simulink library "INT_Rail_SetPoint"  (R2016b)
settings: Solver=VariableStepAuto  StartTime=0.0  StopTime=10.0  RelTol=1e-3
settings Model: Creator=dulinggang  LastModifiedBy=dulinggang

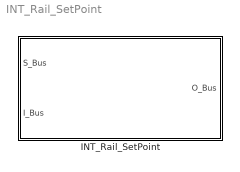
== system INT_Rail_SetPoint ==
  INT_Rail_SetPoint : Subsystem

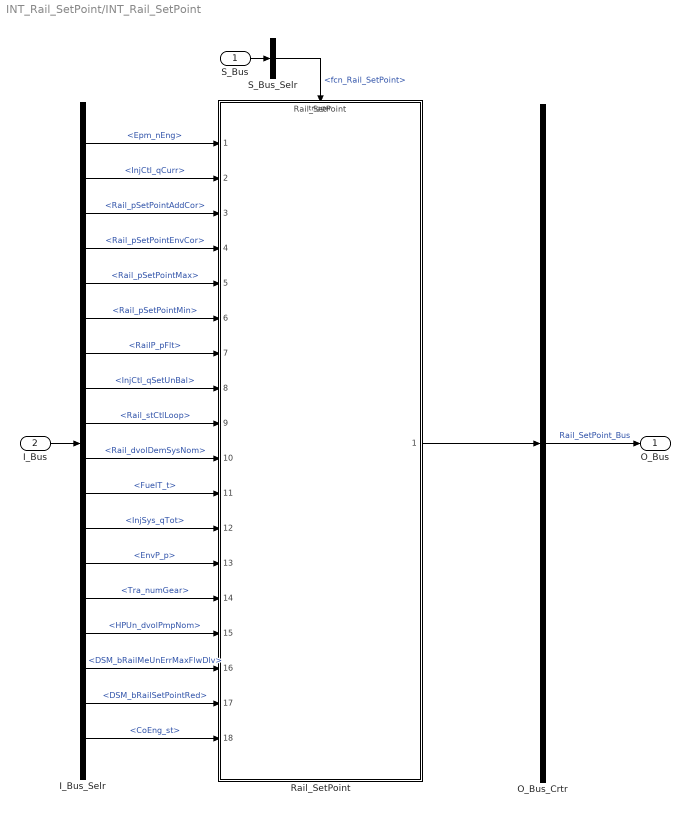
== system INT_Rail_SetPoint/INT_Rail_SetPoint ==
  S_Bus : Inport
  I_Bus : Inport  Port=2
  I_Bus_Selr : BusSelector  OutputSignals=Epm_nEng,InjCtl_qCurr,Rail_pSetPointAddCor,Rail_pSetPointEnvCor,Rail_pSetPointMax,Rail_pSetPointMin,RailP_pFlt,InjCtl_qSetUnBal,Rail_stCtlLoop,Rail_dvolDemSysNom,FuelT_t,InjSys_qTot,EnvP_p,Tra_numGear,HPUn_dvolPmpNom,DSM_bRailMeUnErrMaxFlwDlv,DSM_bRailSetPointRed,CoEng_st
  O_Bus_Crtr : BusCreator  Inputs=1
  Rail_SetPoint : ModelReference  ModelNameDialog=Rail_SetPoint  SimulationMode=Normal  ModelReferenceVersion=1.79  TriggerPortName=function  TriggerPortTriggerType=function-call  TriggerPortStatesWhenEnabling=held
  S_Bus_Selr : BusSelector  OutputSignals=fcn_Rail_SetPoint
  O_Bus : Outport
  wires:
  S_Bus_Selr/1 -> Rail_SetPoint/Trigger  "<fcn_Rail_SetPoint>"
  S_Bus/1 -> S_Bus_Selr/1
  I_Bus/1 -> I_Bus_Selr/1
  I_Bus_Selr/1 -> Rail_SetPoint/1  "<Epm_nEng>"
  I_Bus_Selr/2 -> Rail_SetPoint/2  "<InjCtl_qCurr>"
  I_Bus_Selr/3 -> Rail_SetPoint/3  "<Rail_pSetPointAddCor>"
  I_Bus_Selr/4 -> Rail_SetPoint/4  "<Rail_pSetPointEnvCor>"
  I_Bus_Selr/5 -> Rail_SetPoint/5  "<Rail_pSetPointMax>"
  I_Bus_Selr/6 -> Rail_SetPoint/6  "<Rail_pSetPointMin>"
  I_Bus_Selr/7 -> Rail_SetPoint/7  "<RailP_pFlt>"
  I_Bus_Selr/8 -> Rail_SetPoint/8  "<InjCtl_qSetUnBal>"
  I_Bus_Selr/9 -> Rail_SetPoint/9  "<Rail_stCtlLoop>"
  I_Bus_Selr/10 -> Rail_SetPoint/10  "<Rail_dvolDemSysNom>"
  I_Bus_Selr/11 -> Rail_SetPoint/11  "<FuelT_t>"
  I_Bus_Selr/12 -> Rail_SetPoint/12  "<InjSys_qTot>"
  I_Bus_Selr/13 -> Rail_SetPoint/13  "<EnvP_p>"
  I_Bus_Selr/14 -> Rail_SetPoint/14  "<Tra_numGear>"
  I_Bus_Selr/15 -> Rail_SetPoint/15  "<HPUn_dvolPmpNom>"
  I_Bus_Selr/16 -> Rail_SetPoint/16  "<DSM_bRailMeUnErrMaxFlwDlv>"
  I_Bus_Selr/17 -> Rail_SetPoint/17  "<DSM_bRailSetPointRed>"
  I_Bus_Selr/18 -> Rail_SetPoint/18  "<CoEng_st>"
  O_Bus_Crtr/1 -> O_Bus/1  "Rail_SetPoint_Bus"
  Rail_SetPoint/1 -> O_Bus_Crtr/1
